simulink model "simulink_example_1"  (R2024b)
settings: Solver=VariableStepAuto  StartTime=0.0  StopTime=10.0  RelTol=1e-3
settings Model: Creator=aayus  LastModifiedBy=aayus

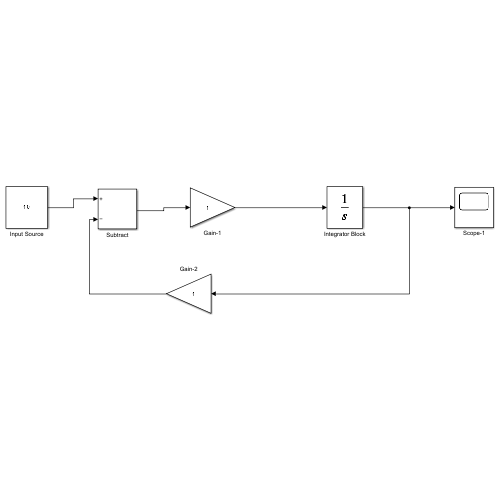
[thumbnail: Simulink's stored preview of the top-level diagram]
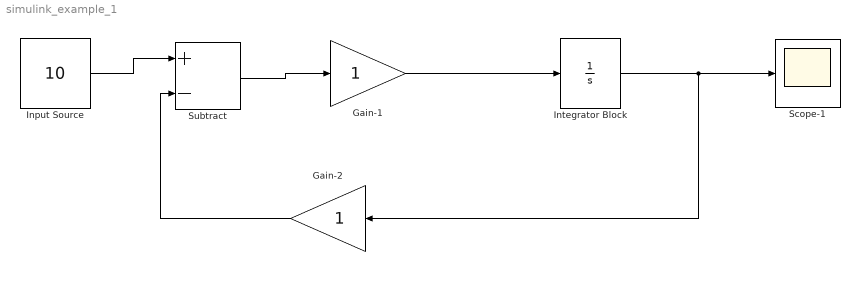
== system simulink_example_1 ==
  Gain-1 : Gain
  Gain-2 : Gain
  Input Source : Constant  Value=10
  Integrator Block : Integrator
  Scope-1 : Scope
  Subtract : Sum  Inputs=+-
  wires:
  Gain-1/1 -> Integrator Block/1
  Integrator Block/1 -> Gain-2/1, Scope-1/1
  Input Source/1 -> Subtract/1
  Subtract/1 -> Gain-1/1
  Gain-2/1 -> Subtract/2
